simulink model "Copy_of_root"  (R2025b)
settings: Solver=VariableStepAuto  StartTime=0.0  StopTime=4  FixedStep=0.001  RelTol=1e-3
settings Model: VariantFading=off  Creator=lew11  LastModifiedBy=rosette-nebula
settings ExplorerConfigSet: InternalSimMechanicsExplorerSettings="<ExplorerConfiguration><canonicalview>default</canonicalview><TilePanel><TileInfo><Tiles Columns=\"1\" Count=\"1\" Height=\"354\" Rows=\"1\" Width=\"500\"><Row Weight=\"1\"/><Column Weight=\"1\"/><Tile Height=\"1\" Width=\"1\" X=\"0\" Y=\"0\"/></Tiles></TileInfo><SceneInfo><SceneViewer><IsThisViewStd><IsStandardView>off</IsStandardView><StandardViewName>Front</StandardViewName></IsThisViewStd><BGColor><R>1</R><G>1</G><B>1</B><A>1</A></BGColor><Camera><DoPerspective>on</DoPerspective><Position><X>58.534417625304727</X><Y>59.860292502851884</Y><Z>-155.4484559381535</Z></Position><Center><X>58.593669358868226</X><Y>61.904700755979775</Y><Z>-155.67104517290912</Z></Center><Up><X>0.0031343571675282087</X><Y>0.10814714230559933</Y><Z>0.99412995700576234</Z></Up><XLim>0.95935498007468478</XLim><YLim>0.95935498007468478</YLim><ViewLimDist>0.01</ViewLimDist></Camera></SceneViewer></SceneInfo></TilePanel><MechEditorPanel><GfxPanelCameraMap><MapElement CameraMLId=\"Camera1\" GfxPanelIndex=\"0\"/></GfxPanelCameraMap><Cameras><Camera><Id>Camera1</Id><Value><Name>Body Cam</Name><NativeCamera><PositionTrackingFeature>Multibody_Sim.Body_Cam.R</PositionTrackingFeature><CenterTrackingFeature>Multibody_Sim.COM_Ref.R</CenterTrackingFeature><UpVectorTrackingFeature>Multibody_Sim.World.W</UpVectorTrackingFeature><CenterTrackingOrigin>on</CenterTrackingOrigin><UpVectorTrackingDirection>+Z</UpVectorTrackingDirection></NativeCamera></Value></Camera><Camera><Id>Camera2</Id><Value><Name>Camera2</Name><NativeCamera><PositionKeyframeSet><Keyframe><Time>0</Time><Value><X>0.11301</X><Y>-1.4589000000000001</Y><Z>0.22284999999999999</Z></Value></Keyframe></PositionKeyframeSet><CenterKeyframeSet><Keyframe><Time>0</Time><Value><X>0.11301</X><Y>-0.55457000000000001</Y><Z>0.22284999999999999</Z></Value></Keyframe></CenterKeyframeSet><UpVectorKeyframeSet><Keyframe><Time>0</Time><Value><X>0</X><Y>0</Y><Z>1</Z></Value></Keyframe></UpVectorKeyframeSet></NativeCamera></Value></Camera><Camera><Id>Camera3</Id><Value><Name>ISO Downwards</Name><NativeCamera><PositionTrackingFeature>Multibody_Sim.TOP.Upper_Structure_Assembly_1_STEP_3_RIGID.F</PositionTrackingFeature><CenterTrackingFeature>Multibody_Sim.Floor_R</CenterTrackingFeature><UpVectorTrackingFeature>Multibody_Sim.Floor_R</UpVectorTrackingFeature><CenterTrackingOrigin>on</CenterTrackingOrigin><UpVectorTrackingDirection>+Z</UpVectorTrackingDirection></NativeCamera></Value></Camera><Camera><Id>Camera4</Id><Value><Name>ISO tracking</Name><NativeCamera><PositionTrackingFeature>Multibody_Sim.World.W</PositionTrackingFeature><CenterTrackingFeature>Multibody_Sim.COM_Ref_R</CenterTrackingFeature><UpVectorTrackingFeature>Multibody_Sim.World_Frame.W</UpVectorTrackingFeature><CenterTrackingOrigin>on</CenterTrackingOrigin><UpVectorTrackingDirection>+Z</UpVectorTrackingDirection></NativeCamera></Value></Camera></Cameras><VideoCreator><IncludeTiles>All</IncludeTiles><IncludeTime>on</IncludeTime><IncludeWorldFrame>off</IncludeWorldFrame><PlaybackSpeedRatio>1</PlaybackSpeedRatio><FrameRate>30</FrameRate><FrameSize>auto</FrameSize><VideoFormat>UncompressedAVI</VideoFormat></VideoCreator></MechEditorPanel><PlaybackSettings><PlaybackSpeedFactor>1</PlaybackSpeedFactor></PlaybackSettings></ExplorerConfiguration>"

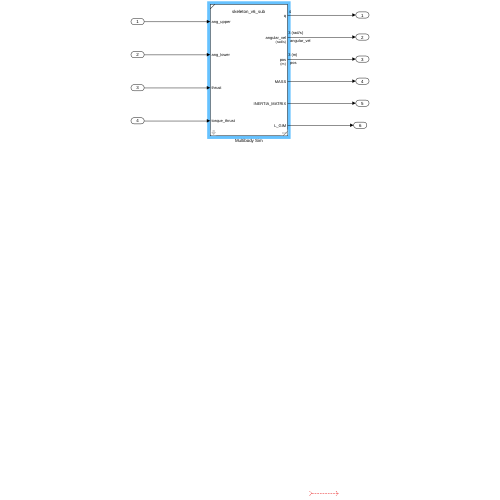
[thumbnail: Simulink's stored preview of the top-level diagram]
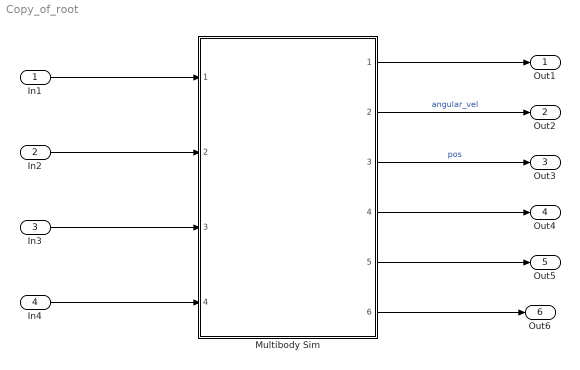
== system Copy_of_root ==
  In1 : Inport
  In2 : Inport  Port=2
  In3 : Inport  Port=3
  In4 : Inport  Port=4
  Multibody Sim : Subsystem  ReferencedSubsystem=skeleton_v6_sub  initial_att=[0,0,0]  initial_ang_vel=[0,0,0]
  Out1 : Outport
  Out2 : Outport  Port=2
  Out3 : Outport  Port=3
  Out4 : Outport  Port=4
  Out5 : Outport  Port=5
  Out6 : Outport  Port=6
  wires:
  ? -> ?
  In1/1 -> Multibody Sim/1
  In2/1 -> Multibody Sim/2
  In3/1 -> Multibody Sim/3
  In4/1 -> Multibody Sim/4
  Multibody Sim/1 -> Out1/1
  Multibody Sim/2 -> Out2/1  "angular_vel"
  Multibody Sim/3 -> Out3/1  "pos"
  Multibody Sim/4 -> Out4/1
  Multibody Sim/5 -> Out5/1
  Multibody Sim/6 -> Out6/1
